simulink model "Copy_of_SWC02_EVP"  (R2020b)
settings: Solver=FixedStepDiscrete  StartTime=0.0  StopTime=10.0  FixedStep=Ts  RelTol=1e-3
model workspace (MAT data in the model file):
  BrkOffPstn = Simulink.Parameter
  BrkOffPstn.Value = 10
  BrkOffPstn.DataType = 'uint8'
  BrkOffPstn.Dimensions = [1 1]
undefined symbols (not defined in the file): IG_On, PrssrDiff_High, PrssrDiff_Low
libraries: simulink x2
settings Model: OrderedModelArguments=off  Creator=Eric  LastModifiedBy=cyw40
settings OptimizationCC: DefaultParameterBehavior=Inlined  EnhancedBackFolding=on  PassReuseOutputArgsAs=Individual arguments  OptimizeBlockOrder=speed  DifferentSizesBufferReuse=on  OptimizationCustomize=off  EfficientTunableParamExpr=on
settings DebuggingCC: ParameterTunabilityLossMsg=error  SFMachineParentedDataDiag=error
settings SFSimCC: MATLABDynamicMemAlloc=off
settings RTWCC: Description=Embedded Coder  SystemTargetFile=ert.tlc  GenCodeOnly=on  TemplateMakefile=ert_default_tmf
settings CodeAppCC: ForceParamTrailComments=on  IgnoreCustomStorageClasses=off  OperatorAnnotations=on  SimulinkDataObjDesc=on  SFDataObjDesc=on  InsertBlockDesc=on
settings ERTTargetCC: TargetLangStandard=C99 (ISO)  GenerateSampleERTMain=on  InlinedParameterPlacement=NonHierarchical  ERTCustomFileTemplate=example_file_process.tlc
settings ConfigComp: DVTestSuiteOptimization=Auto  DVDetectOutOfBounds=on

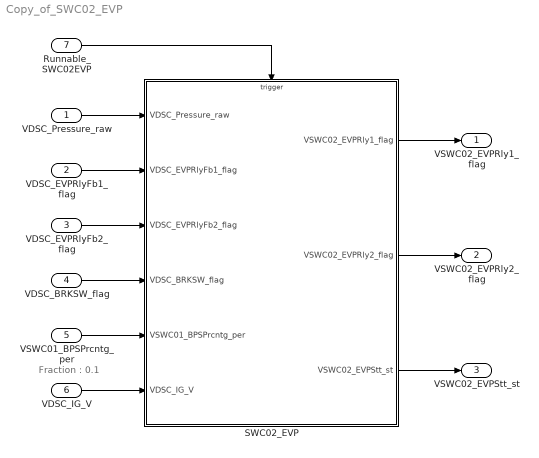
== system Copy_of_SWC02_EVP ==
  note: Fraction : 0.1
  VDSC_Pressure_raw : Inport  OutDataTypeStr=uint16
  VDSC_EVPRlyFb1_flag : Inport  Port=2  OutMin=0  OutMax=1  OutDataTypeStr=boolean
  VDSC_EVPRlyFb2_flag : Inport  Port=3  OutMin=0  OutMax=1  OutDataTypeStr=boolean
  VDSC_BRKSW_flag : Inport  Port=4  OutMin=0  OutMax=1  OutDataTypeStr=boolean  PortDimensions=1
  VSWC01_BPSPrcntg_per : Inport  Port=5  OutMin=0  OutMax=100  OutDataTypeStr=uint8  Unit=%  PortDimensions=1
  VDSC_IG_V : Inport  Port=6  OutMin=0  OutMax=120  OutDataTypeStr=uint8  Unit=V  PortDimensions=1
  Runnable_SWC02EVP : Inport  Port=7  OutputFunctionCall=on
  SWC02_EVP : Subsystem  TreatAsAtomicUnit=on
  VSWC02_EVPRly1_flag : Outport  OutDataTypeStr=boolean
  VSWC02_EVPRly2_flag : Outport  Port=2
  VSWC02_EVPStt_st : Outport  Port=3
  wires:
  Runnable_SWC02EVP/1 -> SWC02_EVP/Trigger
  VDSC_Pressure_raw/1 -> SWC02_EVP/1(VDSC_Pressure_raw)
  SWC02_EVP/1(VSWC02_EVPRly1_flag) -> VSWC02_EVPRly1_flag/1
  SWC02_EVP/3(VSWC02_EVPStt_st) -> VSWC02_EVPStt_st/1
  SWC02_EVP/2(VSWC02_EVPRly2_flag) -> VSWC02_EVPRly2_flag/1
  VDSC_EVPRlyFb2_flag/1 -> SWC02_EVP/3(VDSC_EVPRlyFb2_flag)
  VDSC_EVPRlyFb1_flag/1 -> SWC02_EVP/2(VDSC_EVPRlyFb1_flag)
  VDSC_BRKSW_flag/1 -> SWC02_EVP/4(VDSC_BRKSW_flag)
  VSWC01_BPSPrcntg_per/1 -> SWC02_EVP/5(VSWC01_BPSPrcntg_per)
  VDSC_IG_V/1 -> SWC02_EVP/6(VDSC_IG_V)

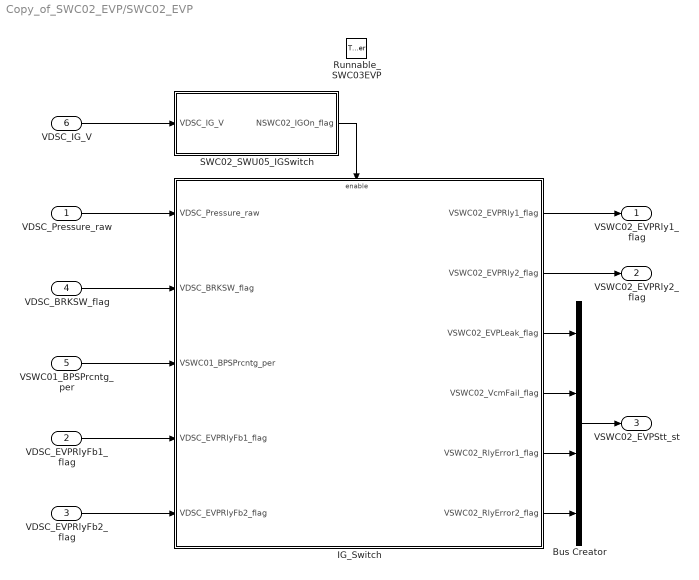
== system Copy_of_SWC02_EVP/SWC02_EVP ==
  VDSC_Pressure_raw : Inport
  VDSC_EVPRlyFb1_flag : Inport  Port=2
  VDSC_EVPRlyFb2_flag : Inport  Port=3
  VDSC_BRKSW_flag : Inport  Port=4
  VSWC01_BPSPrcntg_per : Inport  Port=5
  VDSC_IG_V : Inport  Port=6
  Runnable_SWC03EVP : TriggerPort  TriggerType=function-call  VariantControl=(inherit)
  Bus Creator : BusCreator  Inputs=4
  IG_Switch : Subsystem
  SWC02_SWU05_IGSwitch : Subsystem  TreatAsAtomicUnit=on  RTWFcnName=SWC02_SWU05_IGSwitch
      settings: RTWFcnNameOpts=User specified
  VSWC02_EVPRly1_flag : Outport
  VSWC02_EVPRly2_flag : Outport  Port=2
  VSWC02_EVPStt_st : Outport  Port=3
  wires:
  VDSC_Pressure_raw/1 -> IG_Switch/1(VDSC_Pressure_raw)
  VDSC_BRKSW_flag/1 -> IG_Switch/2(VDSC_BRKSW_flag)
  VSWC01_BPSPrcntg_per/1 -> IG_Switch/3(VSWC01_BPSPrcntg_per)
  VDSC_EVPRlyFb1_flag/1 -> IG_Switch/4(VDSC_EVPRlyFb1_flag)
  VDSC_EVPRlyFb2_flag/1 -> IG_Switch/5(VDSC_EVPRlyFb2_flag)
  IG_Switch/1(VSWC02_EVPRly1_flag) -> VSWC02_EVPRly1_flag/1
  IG_Switch/2(VSWC02_EVPRly2_flag) -> VSWC02_EVPRly2_flag/1
  Bus Creator/1 -> VSWC02_EVPStt_st/1
  VDSC_IG_V/1 -> SWC02_SWU05_IGSwitch/1(VDSC_IG_V)
  SWC02_SWU05_IGSwitch/1(NSWC02_IGOn_flag) -> IG_Switch/Enable
  IG_Switch/3(VSWC02_EVPLeak_flag) -> Bus Creator/1
  IG_Switch/4(VSWC02_VcmFail_flag) -> Bus Creator/2
  IG_Switch/5(VSWC02_RlyError1_flag) -> Bus Creator/3
  IG_Switch/6(VSWC02_RlyError2_flag) -> Bus Creator/4

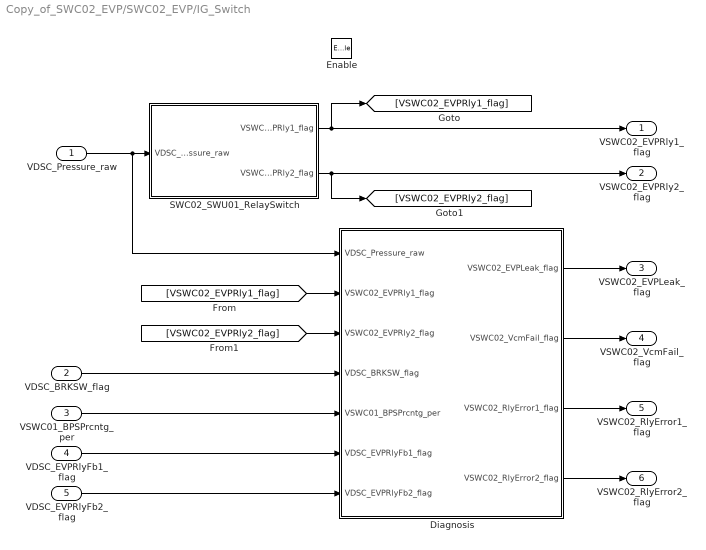
== system Copy_of_SWC02_EVP/SWC02_EVP/IG_Switch ==
  VDSC_Pressure_raw : Inport
  VDSC_BRKSW_flag : Inport  Port=2
  VSWC01_BPSPrcntg_per : Inport  Port=3
  VDSC_EVPRlyFb1_flag : Inport  Port=4
  VDSC_EVPRlyFb2_flag : Inport  Port=5
  Enable : EnablePort  StatesWhenEnabling=reset
  Diagnosis : Subsystem
  SWC02_SWU01_RelaySwitch : Subsystem  TreatAsAtomicUnit=on  RTWFcnName=SWC02_SWU01_RelaySwitch
      settings: RTWFcnNameOpts=User specified
  VSWC02_EVPRly1_flag : Outport  OutputWhenDisabled=reset  InitialOutput=false
  VSWC02_EVPRly2_flag : Outport  Port=2  OutputWhenDisabled=reset  InitialOutput=false
  VSWC02_EVPLeak_flag : Outport  Port=3  OutputWhenDisabled=reset  InitialOutput=false
  VSWC02_VcmFail_flag : Outport  Port=4  OutputWhenDisabled=reset  InitialOutput=false
  VSWC02_RlyError1_flag : Outport  Port=5  OutputWhenDisabled=reset  InitialOutput=false
  VSWC02_RlyError2_flag : Outport  Port=6  OutputWhenDisabled=reset  InitialOutput=false
  wires:
  Diagnosis/2(VSWC02_VcmFail_flag) -> VSWC02_VcmFail_flag/1
  SWC02_SWU01_RelaySwitch/2(VSWC02_EVPRly2_flag) -> VSWC02_EVPRly2_flag/1, [VSWC02_EVPRly2_flag]
  [VSWC02_EVPRly2_flag] -> Diagnosis/3(VSWC02_EVPRly2_flag)
  Diagnosis/4(VSWC02_RlyError2_flag) -> VSWC02_RlyError2_flag/1
  VDSC_Pressure_raw/1 -> SWC02_SWU01_RelaySwitch/1(VDSC_Pressure_raw), Diagnosis/1(VDSC_Pressure_raw)
  Diagnosis/1(VSWC02_EVPLeak_flag) -> VSWC02_EVPLeak_flag/1
  VSWC01_BPSPrcntg_per/1 -> Diagnosis/5(VSWC01_BPSPrcntg_per)
  VDSC_EVPRlyFb1_flag/1 -> Diagnosis/6(VDSC_EVPRlyFb1_flag)
  SWC02_SWU01_RelaySwitch/1(VSWC02_EVPRly1_flag) -> VSWC02_EVPRly1_flag/1, [VSWC02_EVPRly1_flag]
  [VSWC02_EVPRly1_flag] -> Diagnosis/2(VSWC02_EVPRly1_flag)
  Diagnosis/3(VSWC02_RlyError1_flag) -> VSWC02_RlyError1_flag/1
  VDSC_EVPRlyFb2_flag/1 -> Diagnosis/7(VDSC_EVPRlyFb2_flag)
  VDSC_BRKSW_flag/1 -> Diagnosis/4(VDSC_BRKSW_flag)

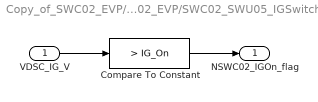
== system Copy_of_SWC02_EVP/SWC02_EVP/SWC02_SWU05_IGSwitch ==
  VDSC_IG_V : Inport
  Compare To Constant : simulink/Logic and Bit Operations/Compare To Constant  relop=>  const=IG_On  OutDataTypeStr=boolean
  NSWC02_IGOn_flag : Outport
  wires:
  VDSC_IG_V/1 -> Compare To Constant/1
  Compare To Constant/1 -> NSWC02_IGOn_flag/1

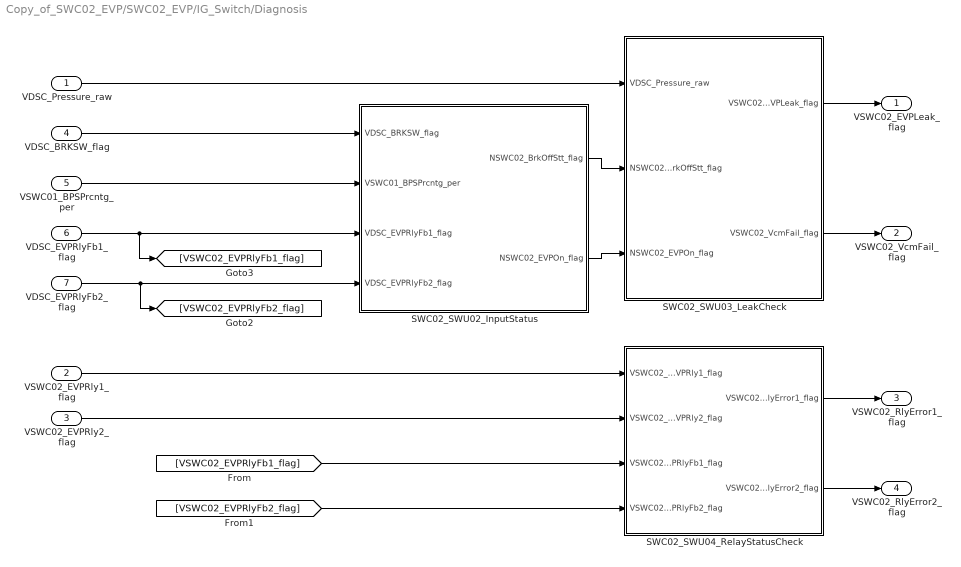
== system Copy_of_SWC02_EVP/SWC02_EVP/IG_Switch/Diagnosis ==
  VDSC_Pressure_raw : Inport
  VSWC02_EVPRly1_flag : Inport  Port=2
  VSWC02_EVPRly2_flag : Inport  Port=3
  VDSC_BRKSW_flag : Inport  Port=4
  VSWC01_BPSPrcntg_per : Inport  Port=5
  VDSC_EVPRlyFb1_flag : Inport  Port=6
  VDSC_EVPRlyFb2_flag : Inport  Port=7
  SWC02_SWU02_InputStatus : Subsystem  TreatAsAtomicUnit=on  RTWFcnName=SWC02_SWU02_InputStatus
      settings: RTWFcnNameOpts=User specified
  SWC02_SWU03_LeakCheck : Subsystem  TreatAsAtomicUnit=on  RTWFcnName=SWC02_SWU03_LeakCheck
      settings: RTWFcnNameOpts=User specified
  SWC02_SWU04_RelayStatusCheck : Subsystem  TreatAsAtomicUnit=on  RTWFcnName=SWC02_SWU04_RelayStatusCheck
      settings: RTWFcnNameOpts=User specified
  VSWC02_EVPLeak_flag : Outport
  VSWC02_VcmFail_flag : Outport  Port=2
  VSWC02_RlyError1_flag : Outport  Port=3
  VSWC02_RlyError2_flag : Outport  Port=4
  wires:
  VDSC_EVPRlyFb1_flag/1 -> [VSWC02_EVPRlyFb1_flag], SWC02_SWU02_InputStatus/3(VDSC_EVPRlyFb1_flag)
  VDSC_EVPRlyFb2_flag/1 -> [VSWC02_EVPRlyFb2_flag], SWC02_SWU02_InputStatus/4(VDSC_EVPRlyFb2_flag)
  VSWC02_EVPRly1_flag/1 -> SWC02_SWU04_RelayStatusCheck/1(VSWC02_EVPRly1_flag)
  VSWC02_EVPRly2_flag/1 -> SWC02_SWU04_RelayStatusCheck/2(VSWC02_EVPRly2_flag)
  [VSWC02_EVPRlyFb1_flag] -> SWC02_SWU04_RelayStatusCheck/3(VSWC02_EVPRlyFb1_flag)
  [VSWC02_EVPRlyFb2_flag] -> SWC02_SWU04_RelayStatusCheck/4(VSWC02_EVPRlyFb2_flag)
  SWC02_SWU04_RelayStatusCheck/1(VSWC02_RlyError1_flag) -> VSWC02_RlyError1_flag/1
  SWC02_SWU04_RelayStatusCheck/2(VSWC02_RlyError2_flag) -> VSWC02_RlyError2_flag/1
  VSWC01_BPSPrcntg_per/1 -> SWC02_SWU02_InputStatus/2(VSWC01_BPSPrcntg_per)
  VDSC_BRKSW_flag/1 -> SWC02_SWU02_InputStatus/1(VDSC_BRKSW_flag)
  SWC02_SWU02_InputStatus/1(NSWC02_BrkOffStt_flag) -> SWC02_SWU03_LeakCheck/2(NSWC02_BrkOffStt_flag)
  VDSC_Pressure_raw/1 -> SWC02_SWU03_LeakCheck/1(VDSC_Pressure_raw)
  SWC02_SWU02_InputStatus/2(NSWC02_EVPOn_flag) -> SWC02_SWU03_LeakCheck/3(NSWC02_EVPOn_flag)
  SWC02_SWU03_LeakCheck/1(VSWC02_EVPLeak_flag) -> VSWC02_EVPLeak_flag/1
  SWC02_SWU03_LeakCheck/2(VSWC02_VcmFail_flag) -> VSWC02_VcmFail_flag/1

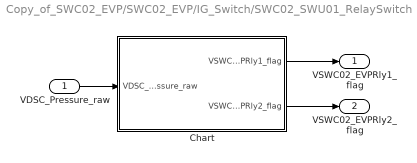
== system Copy_of_SWC02_EVP/SWC02_EVP/IG_Switch/SWC02_SWU01_RelaySwitch ==
  VDSC_Pressure_raw : Inport
  Chart : Stateflow chart  TreatAsAtomicUnit=on
  VSWC02_EVPRly1_flag : Outport
  VSWC02_EVPRly2_flag : Outport  Port=2
  wires:
  Chart/2(VSWC02_EVPRly2_flag) -> VSWC02_EVPRly2_flag/1
  Chart/1(VSWC02_EVPRly1_flag) -> VSWC02_EVPRly1_flag/1
  VDSC_Pressure_raw/1 -> Chart/1(VDSC_Pressure_raw)

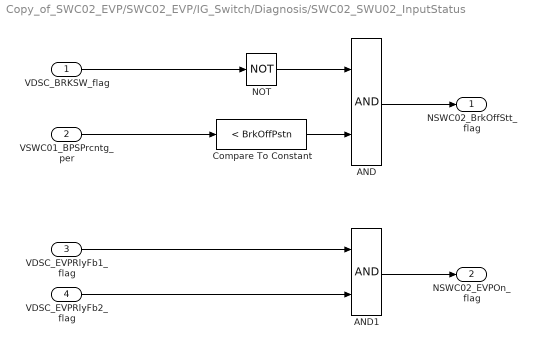
== system Copy_of_SWC02_EVP/SWC02_EVP/IG_Switch/Diagnosis/SWC02_SWU02_InputStatus ==
  VDSC_BRKSW_flag : Inport
  VSWC01_BPSPrcntg_per : Inport  Port=2
  VDSC_EVPRlyFb1_flag : Inport  Port=3
  VDSC_EVPRlyFb2_flag : Inport  Port=4
  AND : Logic  AllPortsSameDT=off  OutDataTypeStr=boolean
  AND1 : Logic  AllPortsSameDT=off  OutDataTypeStr=boolean
  Compare To Constant : simulink/Logic and Bit Operations/Compare To Constant  relop=<  const=BrkOffPstn  OutDataTypeStr=boolean
  NOT : Logic  Operator=NOT  AllPortsSameDT=off  OutDataTypeStr=boolean
  NSWC02_BrkOffStt_flag : Outport
  NSWC02_EVPOn_flag : Outport  Port=2
  wires:
  AND1/1 -> NSWC02_EVPOn_flag/1
  NOT/1 -> AND/1
  AND/1 -> NSWC02_BrkOffStt_flag/1
  VDSC_EVPRlyFb1_flag/1 -> AND1/1
  VSWC01_BPSPrcntg_per/1 -> Compare To Constant/1
  VDSC_EVPRlyFb2_flag/1 -> AND1/2
  VDSC_BRKSW_flag/1 -> NOT/1
  Compare To Constant/1 -> AND/2

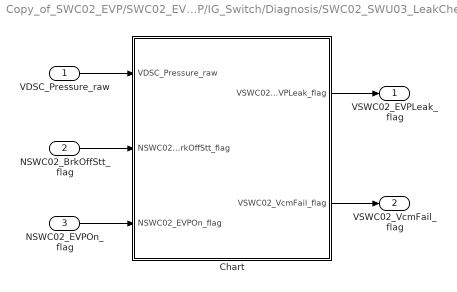
== system Copy_of_SWC02_EVP/SWC02_EVP/IG_Switch/Diagnosis/SWC02_SWU03_LeakCheck ==
  VDSC_Pressure_raw : Inport
  NSWC02_BrkOffStt_flag : Inport  Port=2
  NSWC02_EVPOn_flag : Inport  Port=3
  Chart : Stateflow chart  TreatAsAtomicUnit=on
      settings: PortSchema="{\"entries\":[{\"content\":{\"sides\":[{\"content\":{\"connectorIds\":[\"In2\",\"In1\",\"In3\"]},\"type\":\"ConnectorPlacement.EquallySpacedRectSide\",\"uuid\":\"75a4c2f7-8b67-4ffc-ba2f-7f2deabb0315\"},{\"content\":{\"connectorIds\":[\"Out1\",\"Out2\"],\"side\":\"RIGHT\"},\"type\":\"ConnectorPlacement.EquallySpacedRectSide\",\"uuid\":\"3415e211-2fd3-4410-91fa-3a440a99130d\"},{\"content\":{\"connectorIds\":[],\"side\":\"TOP\"},\"type\":\"ConnectorPlacement.EquallySpacedRectSide\",\"uuid\":\"d91f3903-ebb0-4353-9601-fc8aefc81f12\"}]},\"type\":\"ConnectorPlacement.EquallySpacedConnector\",\"uuid\":\"3dafbae1-cf8d-4072-bd38-ec86ee1d4f95\"}],\"packageUris\":[\"http://schema.mathworks.com/mf0/Connector/R2020b\"],\"version\":\"1.0\"}"
  VSWC02_EVPLeak_flag : Outport
  VSWC02_VcmFail_flag : Outport  Port=2
  wires:
  Chart/1(VSWC02_EVPLeak_flag) -> VSWC02_EVPLeak_flag/1
  Chart/2(VSWC02_VcmFail_flag) -> VSWC02_VcmFail_flag/1
  VDSC_Pressure_raw/1 -> Chart/2(VDSC_Pressure_raw)
  NSWC02_BrkOffStt_flag/1 -> Chart/1(NSWC02_BrkOffStt_flag)
  NSWC02_EVPOn_flag/1 -> Chart/3(NSWC02_EVPOn_flag)

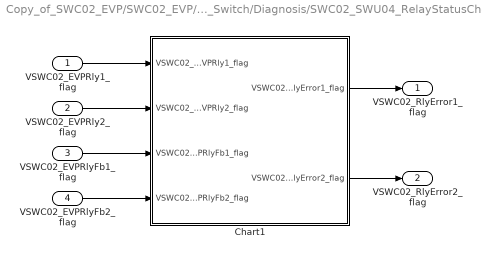
== system Copy_of_SWC02_EVP/SWC02_EVP/IG_Switch/Diagnosis/SWC02_SWU04_RelayStatusCheck ==
  VSWC02_EVPRly1_flag : Inport
  VSWC02_EVPRly2_flag : Inport  Port=2
  VSWC02_EVPRlyFb1_flag : Inport  Port=3
  VSWC02_EVPRlyFb2_flag : Inport  Port=4
  Chart1 : Stateflow chart  TreatAsAtomicUnit=on
  VSWC02_RlyError1_flag : Outport
  VSWC02_RlyError2_flag : Outport  Port=2
  wires:
  VSWC02_EVPRly1_flag/1 -> Chart1/1(VSWC02_EVPRly1_flag)
  Chart1/1(VSWC02_RlyError1_flag) -> VSWC02_RlyError1_flag/1
  VSWC02_EVPRlyFb2_flag/1 -> Chart1/4(VSWC02_EVPRlyFb2_flag)
  Chart1/2(VSWC02_RlyError2_flag) -> VSWC02_RlyError2_flag/1
  VSWC02_EVPRlyFb1_flag/1 -> Chart1/3(VSWC02_EVPRlyFb1_flag)
  VSWC02_EVPRly2_flag/1 -> Chart1/2(VSWC02_EVPRly2_flag)

== stateflow chart Copy_of_SWC02_EVP/SWC02_EVP/IG_Switch/SWC02_SWU01_RelaySwitch/Chart ==
  state Off
    VSWC02_EVPRly1_flag = false;
    VSWC02_EVPRly2_flag = false;
  state On
    VSWC02_EVPRly1_flag = true;
    VSWC02_EVPRly2_flag = true;
  (default) -> Off
  Off -> On : [VDSC_Pressure_raw < PrssrDiff_Low]
  On -> Off : [VDSC_Pressure_raw >= PrssrDiff_High]
  data: VDSC_Pressure_raw input; PrssrDiff_High parameter double; PrssrDiff_Low parameter; VSWC02_EVPRly1_flag output; VSWC02_EVPRly2_flag output

== stateflow chart Copy_of_SWC02_EVP/SWC02_EVP/IG_Switch/Diagnosis/SWC02_SWU03_LeakCheck/Chart ==
  state EVPLeak [parallel]
    settings: executionOrder=1
    state Stop
      First60s = false;
    state Start
      state Check
        (default) -> (junction 25)
        (junction 25) -> (junction 30) [order 1] : [First60s]
        (junction 30) -> (junction 37) [order 1] : [Prssr60s - VDSC_Pressure_raw > 300]
        (junction 25) -> (junction 80) [order 2]
        (junction 30) -> (junction 87) [order 2] : {
            |  VSWC02_EVPLeak_flag = false;
            | }
        (junction 37) -> (junction 44) : {
            |  VSWC02_EVPLeak_flag = true;
            | }
        (junction 87) -> (junction 80)
        (junction 44) -> (junction 87)
        (junction 80) -> (junction 120) : {
            |  Prssr60s = VDSC_Pressure_raw;
            |  First60s = true;
            | }
      state Wait
      (default) -> EVPLeak.Start.Check
      EVPLeak.Start.Check -> EVPLeak.Start.Wait
      EVPLeak.Start.Wait -> EVPLeak.Start.Check : [after(60/Ts -1,tick)]
    (default) -> EVPLeak.Stop
    EVPLeak.Stop -> EVPLeak.Start : [NSWC02_BrkOffStt_flag]
    EVPLeak.Start -> EVPLeak.Stop : [!NSWC02_BrkOffStt_flag]
  state VcmFail [parallel]
    settings: executionOrder=2
    state Stop
      First10s = false;
    state Start
      state Check
        (default) -> (junction 54)
        (junction 54) -> (junction 56) [order 1] : [First10s]
        (junction 56) -> (junction 58) [order 1] : [VDSC_Pressure_raw - Prssr10s < 200]
        (junction 54) -> (junction 84) [order 2]
        (junction 56) -> (junction 74) [order 2] : {
            |  VSWC02_VcmFail_flag = false;
            | }
        (junction 58) -> (junction 72) : {
            |  VSWC02_VcmFail_flag = true;
            | }
        (junction 74) -> (junction 84)
        (junction 72) -> (junction 74)
        (junction 84) -> (junction 170) : {
            |  Prssr10s = VDSC_Pressure_raw;
            |  First10s = true;
            | }
      state Wait
      (default) -> VcmFail.Start.Check
      VcmFail.Start.Check -> VcmFail.Start.Wait
      VcmFail.Start.Wait -> VcmFail.Start.Check : [after(10/Ts -1,tick)]
    (default) -> VcmFail.Stop
    VcmFail.Stop -> VcmFail.Start : [NSWC02_EVPOn_flag]
    VcmFail.Start -> VcmFail.Stop : [!NSWC02_EVPOn_flag]
  data: NSWC02_BrkOffStt_flag input; VDSC_Pressure_raw input; VSWC02_EVPLeak_flag output boolean size=1; NSWC02_EVPOn_flag input; VSWC02_VcmFail_flag output boolean size=1; Prssr10s local uint16 size=1; Prssr60s local uint16 size=1; First10s local boolean size=1; First60s local boolean size=1; Ts parameter

== stateflow chart Copy_of_SWC02_EVP/SWC02_EVP/IG_Switch/Diagnosis/SWC02_SWU04_RelayStatusCheck/Chart1 ==
  state Check
    entry:
    past1 = VSWC02_EVPRly1_flag;
    past2 = VSWC02_EVPRly2_flag;
    on every(0.2/Ts,tick):
    VSWC02_RlyError1_flag = (VSWC02_EVPRlyFb1_flag ~= past1);
    VSWC02_RlyError2_flag = (VSWC02_EVPRlyFb2_flag ~= past2);
    past1 = VSWC02_EVPRly1_flag;
    past2 = VSWC02_EVPRly2_flag;
  (default) -> Check
  data: VSWC02_EVPRly1_flag input; VSWC02_EVPRly2_flag input; VSWC02_EVPRlyFb1_flag input; VSWC02_EVPRlyFb2_flag input; past1 local boolean size=1; VSWC02_RlyError1_flag output; VSWC02_RlyError2_flag output; past2 local boolean size=1; Ts parameter
